simulink library "body_chassis_vert"  (R2018b)
settings: Solver=ode45  StartTime=0.0  StopTime=10.0  RelTol=1e-3  EnableMultiTasking=on
undefined symbols (not defined in the file): DiscIntNeverNeededParam, par_VEH, phi0, psip0, stepsize, v0
libraries: $bdroot x4
(part 1 of 2)
settings Model: Creator=CA-Win7Pro2  LastModifiedBy=ga35gug
settings DataIOCC: LimitDataPoints=on  SaveFormat=Array  SignalLoggingSaveFormat=ModelDataLogs
settings OptimizationCC: LifeSpan=inf
settings DebuggingCC: UnderspecifiedInitializationDetection=Classic  MergeDetectMultiDrivingBlocksExec=none  SolverPrmCheckMsg=warning  MultiTaskDSMMsg=warning  MultiTaskCondExecSysMsg=none  AllowSymbolicDim=off  SFUnexpectedBacktrackingDiag=warning  SFNoUnconditionalDefaultTransitionDiag=warning  SFExecutionAtInitializationDiag=none
settings HardwareCC: ProdBitPerPointer=32  ProdBitPerSizeT=32  ProdBitPerPtrDiffT=32  ProdLargestAtomicFloat=None  ProdIntDivRoundTo=Undefined  ProdEndianess=Unspecified  ProdWordSize=32  ProdHWDeviceType=32-bit Generic
settings ModelReferenceCC: PropagateSignalLabelsOutOfModel=off
settings SFSimCC: SimUseLocalCustomCode=off
settings RTWCC: RTWUseLocalCustomCode=off
settings CodeAppCC: StateflowObjectComments=on
settings GRTTargetCC: TargetLangStandard=C89/C90 (ANSI)  GeneratePreprocessorConditionals=Disable all
settings ConfigComp: CovMetricSettings=dw  CovHtmlReporting=on  CovSaveCumulativeToWorkspaceVar=on  CovSaveSingleToWorkspaceVar=on  CovExternalEMLEnable=off

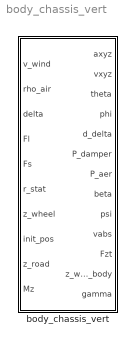
== system body_chassis_vert ==
  body_chassis_vert : Subsystem

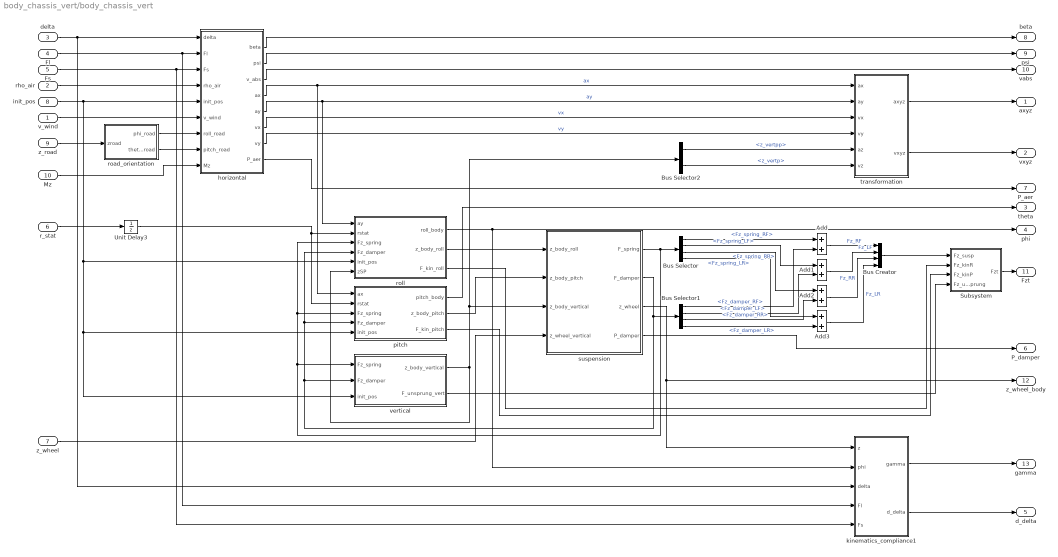
== system body_chassis_vert/body_chassis_vert ==
  v_wind : Inport
  rho_air : Inport  Port=2
  delta : Inport  Port=3
  Fl : Inport  Port=4
  Fs : Inport  Port=5
  r_stat : Inport  Port=6
  z_wheel : Inport  Port=7
  init_pos : Inport  Port=8
  z_road : Inport  Port=9
  Mz : Inport  Port=10
  Add{,1..3} (4 alike) : Sum
  Bus Creator : BusCreator  Inputs=4
  Bus Selector : BusSelector  OutputSignals=Fz_spring_RF,Fz_spring_LF,Fz_spring_RR,Fz_spring_LR
  Bus Selector1 : BusSelector  OutputSignals=Fz_damper_RF,Fz_damper_LF,Fz_damper_RR,Fz_damper_LR
  Bus Selector2 : BusSelector  OutputSignals=z_vertpp,z_vertp
  Subsystem : Subsystem
  Unit Delay3 : UnitDelay  SampleTime=-1
  horizontal : Subsystem
  kinematics_compliance1 : Subsystem
  pitch : Subsystem
  road_orientation : Subsystem
  roll : Subsystem
  suspension : Subsystem
  transformation : Subsystem
  vertical : Subsystem
  axyz : Outport
  vxyz : Outport  Port=2
  theta : Outport  Port=3
  phi : Outport  Port=4
  d_delta : Outport  Port=5
  P_damper : Outport  Port=6
  P_aer : Outport  Port=7
  beta : Outport  Port=8
  psi : Outport  Port=9
  vabs : Outport  Port=10
  Fzt : Outport  Port=11
  z_wheel_body : Outport  Port=12
  gamma : Outport  Port=13
  wires:
  Mz/1 -> horizontal/9(Mz)
  kinematics_compliance1/2(d_delta) -> d_delta/1
  kinematics_compliance1/1(gamma) -> gamma/1
  road_orientation/2(theta_road) -> horizontal/8(pitch_road)
  road_orientation/1(phi_road) -> horizontal/7(roll_road)
  z_road/1 -> road_orientation/1(zroad)
  suspension/3(z_wheel) -> z_wheel_body/1, kinematics_compliance1/1(z)
  roll/1(roll_body) -> phi/1, kinematics_compliance1/2(phi)
  suspension/1(F_spring) -> roll/3(Fz_spring), pitch/3(Fz_spring), vertical/1(Fz_spring), Bus Selector/1
  suspension/2(F_damper) -> roll/4(Fz_damper), pitch/4(Fz_damper), vertical/2(Fz_damper), Bus Selector1/1
  pitch/3(F_kin_pitch) -> Subsystem/3(Fz_kinP)
  roll/3(F_kin_roll) -> Subsystem/2(Fz_kinR)
  Subsystem/1(Fzt) -> Fzt/1
  Bus Creator/1 -> Subsystem/1(Fz_susp)
  pitch/1(pitch_body) -> theta/1
  horizontal/6(vx) -> transformation/3(vx)  "vx"
  horizontal/7(vy) -> transformation/4(vy)  "vy"
  horizontal/5(ay) -> transformation/2(ay), roll/1(ay)  "ay"
  horizontal/4(ax) -> transformation/1(ax), pitch/1(ax)  "ax"
  transformation/1(axyz) -> axyz/1
  transformation/2(vxyz) -> vxyz/1
  Bus Selector2/2 -> transformation/6(vz)  "<z_vertp>"
  Bus Selector2/1 -> transformation/5(az)  "<z_vertpp>"
  Add3/1 -> Bus Creator/4  "Fz_LR"
  Add2/1 -> Bus Creator/3  "Fz_RR"
  Add1/1 -> Bus Creator/2  "Fz_LF"
  Add/1 -> Bus Creator/1  "Fz_RF"
  Bus Selector1/4 -> Add3/2  "<Fz_damper_LR>"
  Bus Selector/4 -> Add3/1  "<Fz_spring_LR>"
  Bus Selector1/3 -> Add2/2  "<Fz_damper_RR>"
  Bus Selector/3 -> Add2/1  "<Fz_spring_RR>"
  Bus Selector1/2 -> Add1/2  "<Fz_damper_LF>"
  Bus Selector/2 -> Add1/1  "<Fz_spring_LF>"
  Bus Selector1/1 -> Add/2  "<Fz_damper_RF>"
  Bus Selector/1 -> Add/1  "<Fz_spring_RF>"
  roll/2(z_body_roll) -> suspension/1(z_body_roll)
  pitch/2(z_body_pitch) -> suspension/2(z_body_pitch)
  z_wheel/1 -> suspension/4(z_wheel_vertical)
  vertical/1(z_body_vertical) -> Bus Selector2/1, suspension/3(z_body_vertical), roll/6(zSP)
  v_wind/1 -> horizontal/6(v_wind)
  init_pos/1 -> horizontal/5(init_pos), pitch/5(init_pos), vertical/3(init_pos), roll/5(init_pos)
  rho_air/1 -> horizontal/4(rho_air)
  Unit Delay3/1 -> pitch/2(rstat), roll/2(rstat)
  delta/1 -> horizontal/1(delta), kinematics_compliance1/3(delta)
  horizontal/1(beta) -> beta/1
  horizontal/2(psi) -> psi/1
  Fl/1 -> horizontal/2(Fl), kinematics_compliance1/4(Fl)
  horizontal/3(v_abs) -> vabs/1
  Fs/1 -> horizontal/3(Fs), kinematics_compliance1/5(Fs)
  r_stat/1 -> Unit Delay3/1
  suspension/4(P_damper) -> P_damper/1
  horizontal/8(P_aer) -> P_aer/1
  vertical/2(F_unsprung_vert) -> Subsystem/4(Fz_unsprung)

== system body_chassis_vert/body_chassis_vert/Subsystem ==
  Fz_susp : Inport
  Fz_kinR : Inport  Port=2
  Fz_kinP : Inport  Port=3
  Fz_unsprung : Inport  Port=4
  Bus Creator : BusCreator  Inputs=4
  Bus Selector : BusSelector  OutputSignals=Fz_RF,Fz_LF,Fz_RR,Fz_LR
  Bus Selector1 : BusSelector  OutputSignals=F_kinR_RF,F_kinR_LF,F_kinR_RR,F_kinR_LR
  Bus Selector2 : BusSelector  OutputSignals=F_kinP_RF,F_kinP_LF,F_kinP_RR,F_kinP_LR
  Bus Selector3 : BusSelector  OutputSignals=F_us_RF,F_us_LF,F_us_RR,F_us_LR
  LF : Sum  Inputs=++++
  LR : Sum  Inputs=++++
  RF : Sum  Inputs=++++
  RR : Sum  Inputs=++++
  Fzt : Outport
  wires:
  Bus Selector2/4 -> LR/3  "<F_kinP_LR>"
  Bus Selector2/3 -> RR/3  "<F_kinP_RR>"
  Bus Creator/1 -> Fzt/1
  LR/1 -> Bus Creator/4  "Fz_LR"
  RR/1 -> Bus Creator/3  "Fz_RR"
  LF/1 -> Bus Creator/2  "Fz_LF"
  RF/1 -> Bus Creator/1  "Fz_RF"
  Bus Selector2/2 -> LF/3  "<F_kinP_LF>"
  Bus Selector2/1 -> RF/3  "<F_kinP_RF>"
  Bus Selector1/4 -> LR/2  "<F_kinR_LR>"
  Bus Selector1/3 -> RR/2  "<F_kinR_RR>"
  Bus Selector1/2 -> LF/2  "<F_kinR_LF>"
  Bus Selector1/1 -> RF/2  "<F_kinR_RF>"
  Bus Selector/4 -> LR/1  "<Fz_LR>"
  Bus Selector/3 -> RR/1  "<Fz_RR>"
  Bus Selector/2 -> LF/1  "<Fz_LF>"
  Bus Selector/1 -> RF/1  "<Fz_RF>"
  Fz_kinP/1 -> Bus Selector2/1
  Fz_kinR/1 -> Bus Selector1/1
  Fz_susp/1 -> Bus Selector/1
  Fz_unsprung/1 -> Bus Selector3/1
  Bus Selector3/1 -> RF/4  "<F_us_RF>"
  Bus Selector3/2 -> LF/4  "<F_us_LF>"
  Bus Selector3/3 -> RR/4  "<F_us_RR>"
  Bus Selector3/4 -> LR/4  "<F_us_LR>"

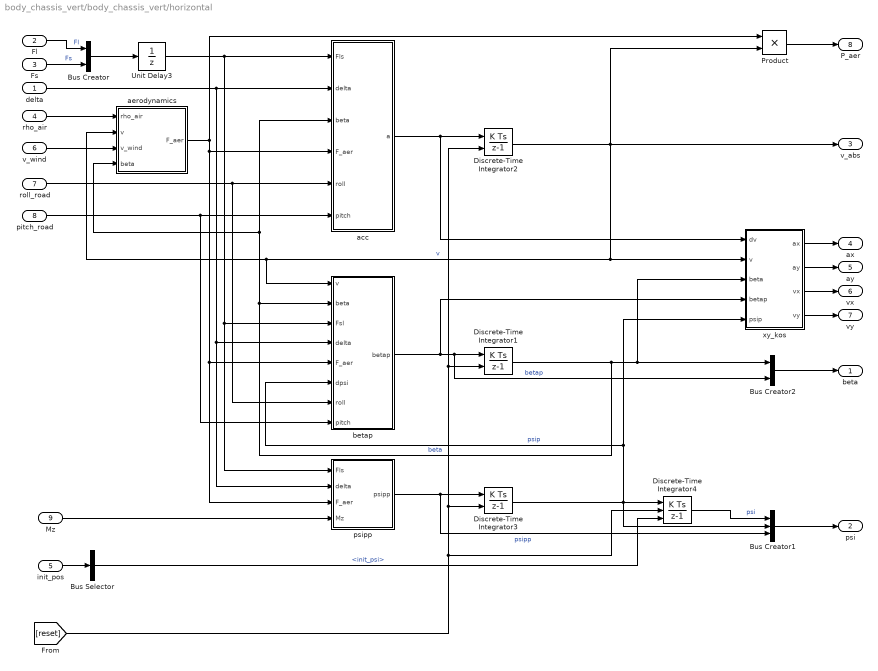
== system body_chassis_vert/body_chassis_vert/horizontal ==
  delta : Inport
  Fl : Inport  Port=2
  Fs : Inport  Port=3
  rho_air : Inport  Port=4
  init_pos : Inport  Port=5
  v_wind : Inport  Port=6
  roll_road : Inport  Port=7
  pitch_road : Inport  Port=8
  Mz : Inport  Port=9
  Bus Creator : BusCreator  Inputs=2
  Bus Creator1 : BusCreator  Inputs=3
  Bus Creator2 : BusCreator  Inputs=2
  Bus Selector : BusSelector  OutputSignals=init_psi
  Discrete-Time Integrator1 : DiscreteIntegrator  ExternalReset=sampled level  SampleTime=-1  ICPrevOutput=DiscIntNeverNeededParam  ICPrevScaledInput=DiscIntNeverNeededParam
  Discrete-Time Integrator2 : DiscreteIntegrator  ExternalReset=sampled level  InitialCondition=v0  SampleTime=-1  ICPrevOutput=DiscIntNeverNeededParam  ICPrevScaledInput=DiscIntNeverNeededParam
  Discrete-Time Integrator3 : DiscreteIntegrator  ExternalReset=sampled level  InitialCondition=psip0  SampleTime=-1  ICPrevOutput=DiscIntNeverNeededParam  ICPrevScaledInput=DiscIntNeverNeededParam
  Discrete-Time Integrator4 : DiscreteIntegrator  ExternalReset=sampled level  InitialConditionSource=external  SampleTime=-1  ICPrevOutput=DiscIntNeverNeededParam  ICPrevScaledInput=DiscIntNeverNeededParam
  Product : Product
  Unit Delay3 : UnitDelay  SampleTime=-1
  acc : Subsystem
  aerodynamics : Subsystem
  betap : Subsystem
  psipp : Subsystem
  xy_kos : Subsystem
  beta : Outport
  psi : Outport  Port=2
  v_abs : Outport  Port=3
  ax : Outport  Port=4
  ay : Outport  Port=5
  vx : Outport  Port=6
  vy : Outport  Port=7
  P_aer : Outport  Port=8
  wires:
  Mz/1 -> psipp/4(Mz)
  Bus Creator2/1 -> beta/1
  pitch_road/1 -> betap/8(pitch), acc/6(pitch)
  roll_road/1 -> acc/5(roll), betap/7(roll)
  xy_kos/4(vy) -> vy/1
  xy_kos/2(ay) -> ay/1
  v_wind/1 -> aerodynamics/3(v_wind)
  Bus Selector/1 -> Discrete-Time Integrator4/3  "<init_psi>"
  init_pos/1 -> Bus Selector/1
  [reset] -> Discrete-Time Integrator4/2, Discrete-Time Integrator3/2, Discrete-Time Integrator1/2, Discrete-Time Integrator2/2
  rho_air/1 -> aerodynamics/1(rho_air)
  xy_kos/1(ax) -> ax/1
  Bus Creator/1 -> Unit Delay3/1
  Fl/1 -> Bus Creator/1  "Fl"
  Fs/1 -> Bus Creator/2  "Fs"
  Discrete-Time Integrator3/1 -> xy_kos/5(psip), betap/6(dpsi), Discrete-Time Integrator4/1, Bus Creator1/2  "psip"
  psipp/1(psipp) -> Discrete-Time Integrator3/1, Bus Creator1/3  "psipp"
  Discrete-Time Integrator1/1 -> xy_kos/3(beta), Bus Creator2/1, aerodynamics/4(beta), acc/3(beta), betap/2(beta)  "beta"
  betap/1(betap) -> xy_kos/4(betap), Discrete-Time Integrator1/1, Bus Creator2/2  "betap"
  delta/1 -> acc/2(delta), psipp/2(delta), betap/4(delta)
  aerodynamics/1(F_aer) -> psipp/3(F_aer), betap/5(F_aer), acc/4(F_aer), Product/1
  Discrete-Time Integrator2/1 -> v_abs/1, Product/2, aerodynamics/2(v), betap/1(v), xy_kos/2(v)  "v"
  acc/1(a) -> xy_kos/1(dv), Discrete-Time Integrator2/1
  Discrete-Time Integrator4/1 -> Bus Creator1/1  "psi"
  Bus Creator1/1 -> psi/1
  xy_kos/3(vx) -> vx/1
  Unit Delay3/1 -> acc/1(Fls), psipp/1(Fls), betap/3(Fsl)
  Product/1 -> P_aer/1

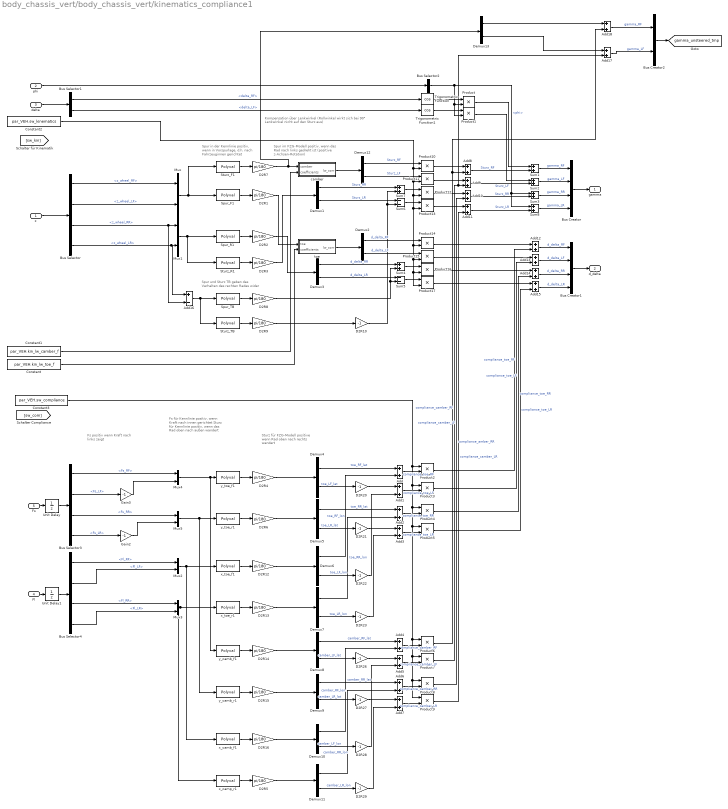
== system body_chassis_vert/body_chassis_vert/kinematics_compliance1 ==
  note: Spur und Sturz TB geben das
      | Verhalten des rechten Rades wider
  note: Spur in der Kennlinie positiv,
      | wenn in Vorspurlage, d.h. nach
      | Fahrzeuginnen gerichtet
  note: Fs für Kennlinie positiv,
      | wenn Kraft nach innen gerichtet
      |
      | Sturz für Kennlinie positiv,
      | wenn das Rad oben nach
      | außen wandert
  note: Fs positiv wenn
      | Kraft nach links zeigt
  note: Kompensation über Lenkwinkel
      | (Rollwinkel wirkt sich bei 90° Lenkwinkel nicht auf den Sturz aus)
  note: Sturz für FZG-Modell
      | positive wenn Rad oben
      | nach rechts wandert
  note: Spur im FZG-Modell positiv,
      | wenn das Rad nach links gedreht ist
      | (positive z-Achsen-Rotation)
  z : Inport
  phi : Inport  Port=2
  delta : Inport  Port=3
  Fl : Inport  Port=4
  Fs : Inport  Port=5
  Add{,1..15,17..18} (18 alike) : Sum
  Add16 : Sum  Inputs=+-
  Bus Creator : BusCreator  Inputs=4
  Bus Creator1 : BusCreator  Inputs=4
  Bus Creator2 : BusCreator  Inputs=2
  Bus Selector : BusSelector  OutputSignals=z_wheel_RF,z_wheel_LF,z_wheel_RR,z_wheel_LR
  Bus Selector1 : BusSelector  OutputSignals=delta_RF,delta_LF
  Bus Selector2 : BusSelector  OutputSignals=phi
  Bus Selector3 : BusSelector  OutputSignals=Fs_RF,Fs_LF,Fs_RR,Fs_LR
  Bus Selector4 : BusSelector  OutputSignals=Fl_RF,Fl_LF,Fl_RR,Fl_LR
  Constant : Constant  Value=par_VEH.kin_lw_toe_f
  Constant1 : Constant  Value=par_VEH.kin_lw_camber_f
  Constant2 : Constant  Value=par_VEH.sw_kinematics
  Constant3 : Constant  Value=par_VEH.sw_compliance
  D2R{1..9,12..16} (14 alike) : Gain  Gain=pi/180
  D2R{10,20..23,26..29} (9 alike) : Gain  Gain=-1
  Demux{1..13} (13 alike) : Demux  Outputs=2
  Gain2 : Gain  Gain=-1
  Gain3 : Gain  Gain=-1
  Mux{,1..5} (6 alike) : Mux  Inputs=2
  Product{,1..17} (18 alike) : Product  RndMeth=Zero
  Spur_F1 : Polyval  Coefs=par_VEH.kin_toe_f
  Spur_R1 : Polyval  Coefs=par_VEH.kin_toe_r
  Spur_TB : Polyval  Coefs=par_VEH.elkin_toe_twistbeam
  Sturz_F1 : Polyval  Coefs=par_VEH.kin_camb_f
  Sturz_R1 : Polyval  Coefs=par_VEH.kin_camb_r
  Sturz_TB : Polyval  Coefs=par_VEH.elkin_camb_twistbeam
  Sum{1..4,7..8} (6 alike) : Sum
  Sum5 : Sum  Inputs=--
  Sum6 : Sum  Inputs=--
  Trigonometric Function : Trigonometry  Operator=cos
  Trigonometric Function1 : Trigonometry  Operator=cos
  Unit Delay : UnitDelay  SampleTime=-1
  Unit Delay1 : UnitDelay  SampleTime=-1
  camber : Subsystem
  toe : Subsystem
  x_camb_f1 : Polyval  Coefs=par_VEH.elkin_x_camb_f
  x_camp_r1 : Polyval  Coefs=par_VEH.elkin_x_camb_r
  x_toe_f1 : Polyval  Coefs=par_VEH.elkin_x_toe_f
  x_toe_r1 : Polyval  Coefs=par_VEH.elkin_x_toe_r
  y_camb_f1 : Polyval  Coefs=par_VEH.elkin_y_camb_f
  y_camb_r1 : Polyval  Coefs=par_VEH.elkin_y_camb_r
  y_toe_f1 : Polyval  Coefs=par_VEH.elkin_y_toe_f
  y_toe_r1 : Polyval  Coefs=par_VEH.elkin_y_toe_r
  gamma : Outport
  d_delta : Outport  Port=2
  tag scope: gamma_unsteered_tmp=global
  wires:
  Bus Creator2/1 -> [gamma_unsteered_tmp]
  Add17/1 -> Bus Creator2/2  "gamma_LF"
  Add18/1 -> Bus Creator2/1  "gamma_RF"
  Demux13/1 -> Add18/1
  Demux13/2 -> Add17/1
  Constant1/1 -> camber/2(coefficients)
  Constant/1 -> toe/2(coefficients)
  D2R1/1 -> toe/1("toe ")
  toe/1(lw_corr) -> Demux2/1
  camber/1(lw_corr) -> Demux12/1
  Mux1/1 -> Sturz_R1/1, Spur_R1/1
  Spur_R1/1 -> D2R2/1
  Spur_F1/1 -> D2R1/1
  Sturz_F1/1 -> D2R7/1
  D2R7/1 -> camber/1("camber "), Demux13/1
  Mux/1 -> Sturz_F1/1, Spur_F1/1
  y_toe_f1/1 -> D2R4/1
  y_toe_r1/1 -> D2R6/1
  x_toe_f1/1 -> D2R12/1
  x_toe_r1/1 -> D2R13/1
  y_camb_f1/1 -> D2R14/1
  y_camb_r1/1 -> D2R15/1
  x_camb_f1/1 -> D2R16/1
  x_camp_r1/1 -> D2R5/1
  D2R3/1 -> Demux1/1
  Demux2/1 -> Product14/1  "d_delta_RF"
  Demux3/1 -> Sum4/1  "d_delta_RR"
  Add7/1 -> Product9/2  "compliance_camber_LR"
  Add6/1 -> Product8/2  "compliance_camber_RR"
  Add5/1 -> Product7/2  "compliance_camber_LF"
  Add4/1 -> Product6/2  "compliance_camber_RF"
  Add3/1 -> Product5/2  "compliance_toe_LR"
  Add2/1 -> Product4/2  "compliance_toe_RR"
  Add1/1 -> Product3/2  "compliance_toe_LF"
  Add/1 -> Product2/2  "compliance_toe_RF"
  Add13/1 -> Bus Creator1/2  "d_delta_LF"
  Unit Delay1/1 -> Bus Selector4/1
  Unit Delay/1 -> Bus Selector3/1
  Fs/1 -> Unit Delay/1
  Fl/1 -> Unit Delay1/1
  Bus Selector3/1 -> Mux4/1  "<Fs_RF>"
  Bus Selector3/2 -> Gain3/1  "<Fs_LF>"
  Bus Selector3/3 -> Mux5/1  "<Fs_RR>"
  Bus Selector3/4 -> Gain2/1  "<Fs_LR>"
  Bus Selector4/1 -> Mux2/1  "<Fl_RF>"
  Bus Selector4/2 -> Mux2/2  "<Fl_LF>"
  Bus Selector4/3 -> Mux3/1  "<Fl_RR>"
  Bus Selector4/4 -> Mux3/2  "<Fl_LR>"
  Mux2/1 -> x_toe_f1/1, x_camb_f1/1
  Mux3/1 -> x_camp_r1/1, x_toe_r1/1
  Mux4/1 -> y_toe_f1/1, y_camb_f1/1
  Mux5/1 -> y_toe_r1/1, y_camb_r1/1
  D2R4/1 -> Demux4/1
  D2R6/1 -> Demux5/1
  D2R12/1 -> Demux6/1
  D2R13/1 -> Demux7/1
  D2R14/1 -> Demux8/1
  D2R15/1 -> Demux9/1
  D2R16/1 -> Demux10/1
  D2R5/1 -> Demux11/1
  Demux4/1 -> Add/1  "toe_RF_lat"
  Demux4/2 -> D2R20/1  "toe_LF_lat"
  Demux5/1 -> Add2/1  "toe_RR_lat"
  Demux5/2 -> D2R21/1  "toe_LR_lat"
  Demux6/1 -> Add/2  "toe_RF_lon"
  Demux6/2 -> D2R22/1  "toe_LF_lon"
  Demux7/1 -> Add2/2  "toe_RR_lon"
  Demux7/2 -> D2R23/1  "toe_LR_lon"
  Demux8/1 -> Add4/1  "camber_RF_lat"
  Demux8/2 -> D2R26/1  "camber_LF_lat"
  Demux9/1 -> Add6/1  "camber_RR_lat"
  Demux9/2 -> D2R27/1  "camber_LR_lat"
  Demux10/1 -> Add4/2  "camber_RF_lon"
  Demux10/2 -> D2R28/1  "camber_LF_lon"
  Demux11/1 -> Add6/2  "camber_RR_lon"
  Demux11/2 -> D2R29/1  "camber_LR_lon"
  delta/1 -> Bus Selector1/1
  Demux1/2 -> Sum6/1  "Sturz_LR"
  D2R2/1 -> Demux3/1
  Bus Creator1/1 -> d_delta/1
  Bus Creator/1 -> gamma/1
  Demux12/2 -> Product11/1  "Sturz_LF"
  Sturz_R1/1 -> D2R3/1
  z/1 -> Bus Selector/1
  phi/1 -> Bus Selector2/1
  Bus Selector2/1 -> Product1/2, Product/2, Sum3/1, Sum8/1  "<phi>"
  Gain2/1 -> Mux5/2
  D2R20/1 -> Add1/1
  D2R21/1 -> Add3/1
  D2R23/1 -> Add3/2
  Spur_TB/1 -> D2R8/1
  Demux3/2 -> Sum5/1  "d_delta_LR"
  Add16/1 -> Spur_TB/1, Sturz_TB/1
  Sturz_TB/1 -> D2R9/1
  Demux1/1 -> Sum7/1  "Sturz_RR"
  D2R9/1 -> D2R10/1
  D2R10/1 -> Sum6/2, Sum7/2
  D2R8/1 -> Sum5/2, Sum4/2
  Constant3/1 -> Product9/1, Product8/1, Product7/1, Product6/1, Product5/1, Product4/1, Product3/1, Product2/1
  Bus Selector/1 -> Mux/1  "<z_wheel_RF>"
  Bus Selector/2 -> Mux/2  "<z_wheel_LF>"
  Bus Selector/3 -> Add16/2, Mux1/1  "<z_wheel_RR>"
  Bus Selector/4 -> Mux1/2, Add16/1  "<z_wheel_LR>"
  Add9/1 -> Sum2/2  "Sturz_LF"
  Trigonometric Function1/1 -> Product1/1
  Trigonometric Function/1 -> Product/1
  Product/1 -> Sum1/1
  Product1/1 -> Sum2/1
  Add10/1 -> Sum3/2  "Sturz_RR"
  Add11/1 -> Sum8/2  "Sturz_LR"
  Sum8/1 -> Bus Creator/4  "gamma_LR"
  Sum3/1 -> Bus Creator/3  "gamma_RR"
  Sum2/1 -> Bus Creator/2  "gamma_LF"
  Sum1/1 -> Bus Creator/1  "gamma_RF"
  Demux12/1 -> Product10/1  "Sturz_RF"
  Sum6/1 -> Product13/1
  Demux2/2 -> Product15/1  "d_delta_LF"
  Sum4/1 -> Product16/1
  Sum5/1 -> Product17/1
  Constant2/1 -> Product14/2, Product15/2, Product17/2, Product16/2, Product13/2, Product12/2, Product11/2, Product10/2
  Product10/1 -> Add8/1
  Product11/1 -> Add9/1
  Product12/1 -> Add10/1
  Product13/1 -> Add11/1
  Product14/1 -> Add12/1
  Product15/1 -> Add13/1
  Product16/1 -> Add14/1
  Product17/1 -> Add15/1
  Add15/1 -> Bus Creator1/4  "d_delta_LR"
  Add12/1 -> Bus Creator1/1  "d_delta_RF"
  Add14/1 -> Bus Creator1/3  "d_delta_RR"
  Gain3/1 -> Mux4/2
  Add8/1 -> Sum1/2  "Sturz_RF"
  Product2/1 -> Add12/2  "compliance_toe_RF"
  Product3/1 -> Add13/2  "compliance_toe_LF"
  Product4/1 -> Add14/2  "compliance_toe_RR"
  Product5/1 -> Add15/2  "compliance_toe_LR"
  Product6/1 -> Add8/2, Add18/2  "compliance_camber_RF"
  Product7/1 -> Add9/2, Add17/2  "compliance_camber_LF"
  Product8/1 -> Add10/2  "compliance_amber_RR"
  Product9/1 -> Add11/2  "compliance_camber_LR"
  D2R22/1 -> Add1/2
  Bus Selector1/2 -> Trigonometric Function1/1  "<delta_LF>"
  Bus Selector1/1 -> Trigonometric Function/1  "<delta_RF>"
  Sum7/1 -> Product12/1
  D2R26/1 -> Add5/1
  D2R27/1 -> Add7/1
  D2R28/1 -> Add5/2
  D2R29/1 -> Add7/2

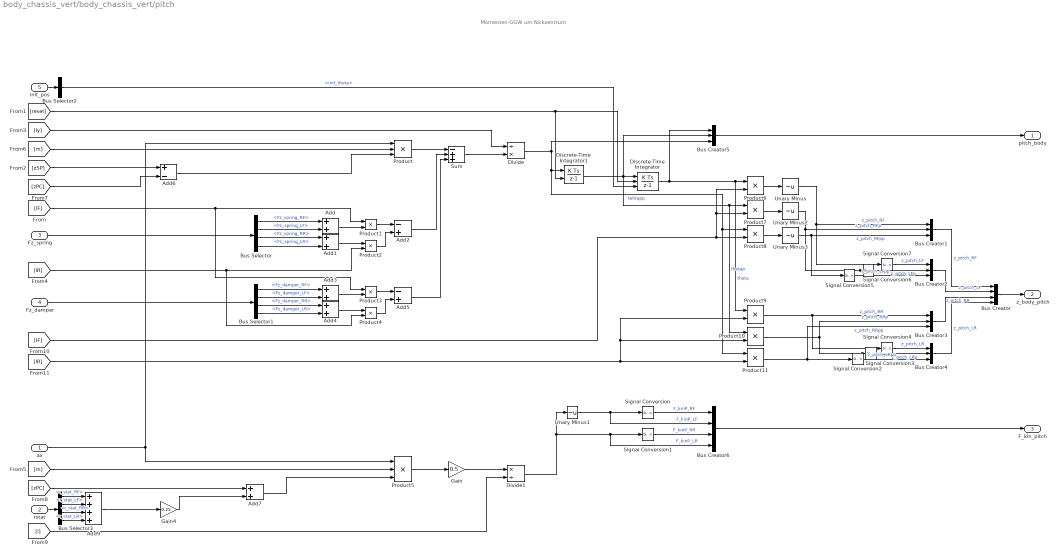
== system body_chassis_vert/body_chassis_vert/pitch ==
  note: Momenten-GGW um Nickzentrum
  ax : Inport
  rstat : Inport  Port=2
  Fz_spring : Inport  Port=3
  Fz_damper : Inport  Port=4
  init_pos : Inport  Port=5
  Add{,1,3..4,7} (5 alike) : Sum
  Add2 : Sum  Inputs=-+
  Add5 : Sum  Inputs=-+
  Add6 : Sum  Inputs=+-
  Add9 : Sum  Inputs=++++
  Bus Creator : BusCreator  Inputs=4
  Bus Creator{1..5} (5 alike) : BusCreator  Inputs=3
  Bus Creator6 : BusCreator  Inputs=4
  Bus Selector : BusSelector  OutputSignals=Fz_spring_RF,Fz_spring_LF,Fz_spring_RR,Fz_spring_LR
  Bus Selector1 : BusSelector  OutputSignals=Fz_damper_RF,Fz_damper_LF,Fz_damper_RR,Fz_damper_LR
  Bus Selector2 : BusSelector  OutputSignals=init_theta
  Bus Selector3 : BusSelector  OutputSignals=r_stat_RF,r_stat_LF,r_stat_RR,r_stat_LR
  Discrete-Time Integrator : DiscreteIntegrator  ExternalReset=sampled level  InitialConditionSource=external  SampleTime=stepsize  ICPrevOutput=DiscIntNeverNeededParam  ICPrevScaledInput=DiscIntNeverNeededParam
  Discrete-Time Integrator1 : DiscreteIntegrator  ExternalReset=sampled level  SampleTime=stepsize  ICPrevOutput=DiscIntNeverNeededParam  ICPrevScaledInput=DiscIntNeverNeededParam
  Divide : Product  Inputs=/*
  Divide1 : Product  Inputs=*/
  Gain : Gain  Gain=0.5
  Gain4 : Gain  Gain=0.25
  Product : Product  Inputs=3  RndMeth=Zero
  Product{1..4,6..11} (10 alike) : Product  RndMeth=Zero
  Product5 : Product  Inputs=3  RndMeth=Zero
  Signal Conversion{,1..7} (8 alike) : SignalConversion  OverrideOpt=off
  Sum : Sum  Inputs=-++
  Unary Minus{,1..3} (4 alike) : UnaryMinus
  pitch_body : Outport
  z_body_pitch : Outport  Port=2
  F_kin_pitch : Outport  Port=3
  wires:
  Unary Minus1/1 -> Signal Conversion/1, Bus Creator6/2  "F_kinP_LF"
  ax/1 -> Product/1, Product5/1
  Divide1/1 -> Unary Minus1/1, Bus Creator6/4, Signal Conversion1/1  "F_kinP_LR"
  Signal Conversion7/1 -> Bus Creator2/1  "z_pitch_LF"
  Signal Conversion6/1 -> Bus Creator2/2  "z_pitch_LFp"
  Signal Conversion5/1 -> Bus Creator2/3  "z_pitch_LFpp"
  Signal Conversion4/1 -> Bus Creator4/1  "z_pitch_LR"
  Signal Conversion3/1 -> Bus Creator4/2  "z_pitch_LRp"
  Signal Conversion2/1 -> Bus Creator4/3  "z_pitch_LRpp"
  Gain4/1 -> Add7/2
  rstat/1 -> Bus Selector3/1
  Bus Selector3/4 -> Add9/4  "<r_stat_LR>"
  Bus Selector3/3 -> Add9/3  "<r_stat_RR>"
  Bus Selector3/2 -> Add9/2  "<r_stat_LF>"
  Bus Selector3/1 -> Add9/1  "<r_stat_RF>"
  Add9/1 -> Gain4/1
  [zPC] -> Add7/1
  [zPC] -> Add6/2
  [zSP] -> Add6/1
  [reset] -> Discrete-Time Integrator/2, Discrete-Time Integrator1/2
  Bus Selector2/1 -> Discrete-Time Integrator/3  "<init_theta>"
  init_pos/1 -> Bus Selector2/1
  Bus Creator/1 -> z_body_pitch/1
  Bus Creator1/1 -> Bus Creator/1  "z_pitch_RF"
  Bus Creator2/1 -> Bus Creator/2  "z_pitch_LF"
  Bus Creator3/1 -> Bus Creator/3  "z_pitch_RR"
  Bus Creator4/1 -> Bus Creator/4  "z_pitch_LR"
  Unary Minus2/1 -> Bus Creator1/2, Signal Conversion6/1  "z_pitch_RFp"
  Discrete-Time Integrator/1 -> Bus Creator5/1, Product9/1, Product6/1  "theta"
  Bus Creator5/1 -> pitch_body/1
  [m] -> Product/2
  Sum/1 -> Divide/2
  [Iy] -> Divide/1
  Divide/1 -> Product8/1, Product11/1, Discrete-Time Integrator1/1, Bus Creator5/3  "tehtapp"
  Discrete-Time Integrator1/1 -> Discrete-Time Integrator/1, Product10/1, Product7/1, Bus Creator5/2  "thetap"
  Fz_spring/1 -> Bus Selector/1
  Bus Selector/1 -> Add/1  "<Fz_spring_RF>"
  Bus Selector/2 -> Add/2  "<Fz_spring_LF>"
  Bus Selector/3 -> Add1/1  "<Fz_spring_RR>"
  Bus Selector/4 -> Add1/2  "<Fz_spring_LR>"
  Fz_damper/1 -> Bus Selector1/1
  Add/1 -> Product1/2
  Add1/1 -> Product2/1
  Product1/1 -> Add2/1
  Product2/1 -> Add2/2
  Bus Selector1/1 -> Add3/1  "<Fz_damper_RF>"
  Bus Selector1/2 -> Add3/2  "<Fz_damper_LF>"
  Bus Selector1/3 -> Add4/1  "<Fz_damper_RR>"
  Bus Selector1/4 -> Add4/2  "<Fz_damper_LR>"
  Add3/1 -> Product3/2
  Add4/1 -> Product4/1
  Product3/1 -> Add5/1
  Product4/1 -> Add5/2
  Unary Minus/1 -> Bus Creator1/1, Signal Conversion7/1  "z_pitch_RF"
  Unary Minus3/1 -> Signal Conversion5/1, Bus Creator1/3  "z_pitch_RFpp"
  Add6/1 -> Product/3
  Product/1 -> Sum/1
  Add5/1 -> Sum/3
  Add2/1 -> Sum/2
  Add7/1 -> Product5/3
  Product5/1 -> Gain/1
  [l] -> Divide1/2
  Gain/1 -> Divide1/1
  Signal Conversion1/1 -> Bus Creator6/3  "F_kinP_RR"
  Bus Creator6/1 -> F_kin_pitch/1
  [m] -> Product5/2
  Signal Conversion/1 -> Bus Creator6/1  "F_kinP_RF"
  [lR] -> Product2/2, Product4/2
  [lF] -> Product1/1, Product3/1
  [lF] -> Product8/2, Product7/2, Product6/2
  [lR] -> Product9/2, Product10/2, Product11/2
  Product9/1 -> Signal Conversion4/1, Bus Creator3/1  "z_pitch_RR"
  Product10/1 -> Signal Conversion3/1, Bus Creator3/2  "z_pitch_RRp"
  Product11/1 -> Signal Conversion2/1, Bus Creator3/3  "z_pitch_RRpp"
  Product8/1 -> Unary Minus3/1
  Product6/1 -> Unary Minus/1
  Product7/1 -> Unary Minus2/1

== system body_chassis_vert/body_chassis_vert/road_orientation ==
  zroad : Inport
  Bus Selector1 : BusSelector  OutputSignals=zroad_RF,zroad_LF,zroad_RR,zroad_LR
  Divide7 : Product  Inputs=*/
  Divide8 : Product  Inputs=*/
  Gain{,1..4} (5 alike) : Gain  Gain=0.5
  Subtract{14..15,17..19} (5 alike) : Sum
  Subtract16 : Sum  Inputs=-+
  Subtract20 : Sum  Inputs=+-
  Trigonometric Function : Trigonometry  Operator=asin
  Trigonometric Function1 : Trigonometry  Operator=asin
  phi_road : Outport
  theta_road : Outport  Port=2
  wires:
  Divide8/1 -> Trigonometric Function/1
  [l] -> Divide8/2
  Subtract20/1 -> Divide8/1
  Gain4/1 -> Subtract20/2
  Gain3/1 -> Subtract20/1
  Subtract19/1 -> Gain4/1
  Subtract18/1 -> Gain3/1
  Bus Selector1/1 -> Subtract14/1, Subtract18/1  "<zroad_RF>"
  Trigonometric Function/1 -> theta_road/1
  Divide7/1 -> Trigonometric Function1/1
  Subtract17/1 -> Gain2/1
  Gain2/1 -> Divide7/2
  Subtract16/1 -> Divide7/1
  Gain1/1 -> Subtract16/2
  Gain/1 -> Subtract16/1
  Bus Selector1/4 -> Subtract15/2, Subtract19/2  "<zroad_LR>"
  Bus Selector1/2 -> Subtract15/1, Subtract18/2  "<zroad_LF>"
  Subtract15/1 -> Gain1/1
  Bus Selector1/3 -> Subtract14/2, Subtract19/1  "<zroad_RR>"
  [sR] -> Subtract17/1
  Subtract14/1 -> Gain/1
  Trigonometric Function1/1 -> phi_road/1
  [sF] -> Subtract17/2
  zroad/1 -> Bus Selector1/1

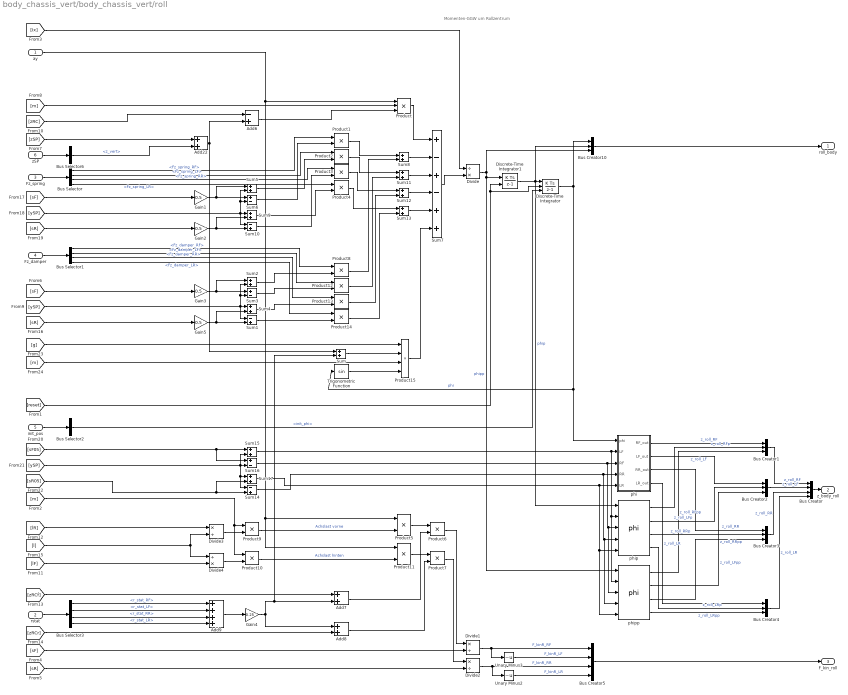
== system body_chassis_vert/body_chassis_vert/roll ==
  note: Momenten-GGW um Rollzentrum
  ay : Inport
  rstat : Inport  Port=2
  Fz_spring : Inport  Port=3
  Fz_damper : Inport  Port=4
  init_pos : Inport  Port=5
  zSP : Inport  Port=6
  Add22 : Sum
  Add6 : Sum  Inputs=-+
  Add7 : Sum
  Add8 : Sum
  Add9 : Sum  Inputs=++++
  Bus Creator : BusCreator  Inputs=4
  Bus Creator{1..4,10} (5 alike) : BusCreator  Inputs=3
  Bus Creator5 : BusCreator  Inputs=4
  Bus Selector : BusSelector  OutputSignals=Fz_spring_RF,Fz_spring_LF,Fz_spring_RR,Fz_spring_LR
  Bus Selector1 : BusSelector  OutputSignals=Fz_damper_RF,Fz_damper_LF,Fz_damper_RR,Fz_damper_LR
  Bus Selector2 : BusSelector  OutputSignals=init_phi
  Bus Selector3 : BusSelector  OutputSignals=r_stat_RF,r_stat_LF,r_stat_RR,r_stat_LR
  Bus Selector6 : BusSelector  OutputSignals=z_vert
  Discrete-Time Integrator : DiscreteIntegrator  ExternalReset=sampled level  InitialConditionSource=external  InitialCondition=phi0  SampleTime=stepsize  ICPrevOutput=DiscIntNeverNeededParam  ICPrevScaledInput=DiscIntNeverNeededParam
  Discrete-Time Integrator1 : DiscreteIntegrator  ExternalReset=sampled level  SampleTime=stepsize  ICPrevOutput=DiscIntNeverNeededParam  ICPrevScaledInput=DiscIntNeverNeededParam
  Divide : Product  Inputs=/*
  Divide1 : Product  Inputs=*/
  Divide2 : Product  Inputs=*/
  Divide3 : Product  Inputs=*/
  Divide4 : Product  Inputs=/*
  Gain{1..3,5} (4 alike) : Gain  Gain=0.5
  Gain4 : Gain  Gain=0.25
  Product : Product  Inputs=3  RndMeth=Zero
  Product{1..14} (14 alike) : Product  RndMeth=Zero
  Product15 : Product  Inputs=4
  Sum{,2,4..5,8..9,11..13,15,17} (11 alike) : Sum
  Sum1 : Sum  Inputs=-+
  Sum10 : Sum  Inputs=-+
  Sum14 : Sum  Inputs=-+
  Sum16 : Sum  Inputs=+-
  Sum3 : Sum  Inputs=+-
  Sum6 : Sum  Inputs=+-
  Sum7 : Sum  Inputs=+-+-++
  Trigonometric Function : Trigonometry
  Unary Minus2 : UnaryMinus
  Unary Minus3 : UnaryMinus
  phi : Subsystem
  phip : $bdroot/body_chassis_vert/roll/phi  SystemSampleTime=-1
  phipp : $bdroot/body_chassis_vert/roll/phi  SystemSampleTime=-1
  roll_body : Outport
  z_body_roll : Outport  Port=2
  F_kin_roll : Outport  Port=3
  wires:
  Product15/1 -> Sum7/6
  [m] -> Product15/3
  Trigonometric Function/1 -> Product15/4
  Sum/1 -> Product15/2
  [g] -> Product15/1
  [m] -> Product/2
  Sum17/1 -> phi/5(LR), phipp/5, phip/5
  Sum14/1 -> phipp/4, phip/4, phi/4(RR)
  Sum16/1 -> phi/3(RF), phipp/3, phip/3
  Sum15/1 -> phi/2(LF), phipp/2, phip/2
  [sR05] -> Sum14/2, Sum17/2
  [sF05] -> Sum16/1, Sum15/1
  Product14/1 -> Sum13/2
  Product13/1 -> Sum12/2
  Product12/1 -> Sum11/2
  Product8/1 -> Sum8/2
  Product4/1 -> Sum13/1
  Product3/1 -> Sum12/1
  Product2/1 -> Sum11/1
  Sum1/1 -> Product14/2
  Sum4/1 -> Product13/2
  Sum3/1 -> Product12/2
  Sum2/1 -> Product8/2
  Gain5/1 -> Sum1/2, Sum4/2
  Gain3/1 -> Sum3/1, Sum2/1
  [sR] -> Gain5/1
  [sF] -> Gain3/1
  Unary Minus3/1 -> Bus Creator5/2  "F_kinR_LF"
  Unary Minus2/1 -> Bus Creator5/4  "F_kinR_LR"
  Sum13/1 -> Sum7/5
  Product/1 -> Sum7/1
  Sum12/1 -> Sum7/4
  Sum11/1 -> Sum7/3
  Sum9/1 -> Product4/2
  Sum10/1 -> Product3/2
  Sum5/1 -> Product2/2
  Sum6/1 -> Product1/2
  Gain2/1 -> Sum9/2, Sum10/2
  Gain1/1 -> Sum5/1, Sum6/1
  Fz_damper/1 -> Bus Selector1/1
  Fz_spring/1 -> Bus Selector/1
  [sR] -> Gain2/1
  [sF] -> Gain1/1
  Bus Selector1/4 -> Product14/1  "<Fz_damper_LR>"
  Bus Selector1/3 -> Product13/1  "<Fz_damper_RR>"
  Bus Selector1/2 -> Product12/1  "<Fz_damper_LF>"
  Bus Selector1/1 -> Product8/1  "<Fz_damper_RF>"
  Bus Selector/4 -> Product4/1  "<Fz_spring_LR>"
  Bus Selector/2 -> Product2/1  "<Fz_spring_LF>"
  Bus Selector/3 -> Product3/1  "<Fz_spring_RR>"
  Bus Selector/1 -> Product1/1  "<Fz_spring_RF>"
  Product7/1 -> Divide2/1
  Product6/1 -> Divide1/1
  Gain4/1 -> Add7/2, Sum/2, Add8/1
  Bus Selector3/4 -> Add9/4  "<r_stat_LR>"
  Bus Selector3/3 -> Add9/3  "<r_stat_RR>"
  Bus Selector3/2 -> Add9/2  "<r_stat_LF>"
  Bus Selector3/1 -> Add9/1  "<r_stat_RF>"
  rstat/1 -> Bus Selector3/1
  Bus Selector2/1 -> Discrete-Time Integrator/3  "<init_phi>"
  init_pos/1 -> Bus Selector2/1
  Bus Creator10/1 -> roll_body/1
  Add8/1 -> Product7/2
  Product11/1 -> Product7/1
  Product5/1 -> Product6/1
  Product10/1 -> Product11/2  "Achslast hinten"
  Product9/1 -> Product5/2  "Achslast vorne"
  Divide4/1 -> Product10/2
  Divide3/1 -> Product9/2
  [l] -> Divide4/1, Divide3/2
  [zRCr] -> Add8/2
  [reset] -> Discrete-Time Integrator/2, Discrete-Time Integrator1/2
  Add9/1 -> Gain4/1
  [zRCf] -> Add7/1
  Add22/1 -> Sum/1, Add6/2
  [zRC] -> Add6/1
  Bus Creator/1 -> z_body_roll/1
  Bus Creator1/1 -> Bus Creator/1  "z_roll_RF"
  Bus Creator2/1 -> Bus Creator/2  "z_roll_LF"
  Bus Creator3/1 -> Bus Creator/3  "z_roll_RR"
  Bus Creator4/1 -> Bus Creator/4  "z_roll_LR"
  phi/1(RF_out) -> Bus Creator1/1  "z_roll_RF"
  phip/1 -> Bus Creator1/2  "z_roll_RFp"
  phipp/1 -> Bus Creator1/3  "z_roll_RFpp"
  phi/2(LF_out) -> Bus Creator2/1  "z_roll_LF"
  phip/2 -> Bus Creator2/2  "z_roll_LFp"
  phipp/2 -> Bus Creator2/3  "z_roll_LFpp"
  phi/3(RR_out) -> Bus Creator3/1  "z_roll_RR"
  phip/3 -> Bus Creator3/2  "z_roll_RRp"
  phipp/3 -> Bus Creator3/3  "z_roll_RRpp"
  phi/4(LR_out) -> Bus Creator4/1  "z_roll_LR"
  phip/4 -> Bus Creator4/2  "z_roll_LRp"
  phipp/4 -> Bus Creator4/3  "z_roll_LRpp"
  [Ix] -> Divide/1
  Divide/1 -> Bus Creator10/3, phipp/1, Discrete-Time Integrator1/1  "phipp"
  Discrete-Time Integrator1/1 -> phip/1, Bus Creator10/2, Discrete-Time Integrator/1  "phip"
  [sF] -> Divide1/2
  [sR] -> Divide2/2
  Divide1/1 -> Unary Minus3/1, Bus Creator5/1  "F_kinR_RF"
  Divide2/1 -> Unary Minus2/1, Bus Creator5/3  "F_kinR_RR"
  Bus Creator5/1 -> F_kin_roll/1
  [m] -> Product9/1, Product10/1
  Sum7/1 -> Divide/2
  ay/1 -> Product/1, Product5/1, Product11/1
  Product1/1 -> Sum8/1
  Sum8/1 -> Sum7/2
  [ySP] -> Sum1/1, Sum4/1, Sum3/2, Sum2/2
  [ySP] -> Sum5/2, Sum6/2, Sum9/1, Sum10/1
  [ySP] -> Sum16/2, Sum15/2, Sum14/1, Sum17/1
  Add7/1 -> Product6/2
  zSP/1 -> Bus Selector6/1
  [zSP] -> Add22/1
  Bus Selector6/1 -> Add22/2  "<z_vert>"
  [lR] -> Divide3/1
  [lF] -> Divide4/2
  Discrete-Time Integrator/1 -> Bus Creator10/1, Trigonometric Function/1, phi/1(phi)  "phi"
  Add6/1 -> Product/3

== system body_chassis_vert/body_chassis_vert/suspension ==
  z_body_roll : Inport
  z_body_pitch : Inport  Port=2
  z_body_vertical : Inport  Port=3
  z_wheel_vertical : Inport  Port=4
  Add{,1..3} (4 alike) : Sum
  Bus Creator : BusCreator  Inputs=4
  Bus Selector : BusSelector  OutputSignals=Fz_spring_RF,Fz_spring_LF,Fz_spring_RR,Fz_spring_LR
  Bus Selector1 : BusSelector  OutputSignals=Fz_arb_RF,Fz_arb_LF,Fz_arb_RR,Fz_arb_LR
  arb : Subsystem
  damper : Subsystem
  spring : Subsystem
  F_spring : Outport
  F_damper : Outport  Port=2
  z_wheel : Outport  Port=3
  P_damper : Outport  Port=4
  wires:
  spring/2(z_wheel) -> z_wheel/1
  spring/1(Fz_spring) -> Bus Selector/1
  arb/1(F_arb) -> Bus Selector1/1
  Bus Selector/1 -> Add/1  "<Fz_spring_RF>"
  Bus Selector1/1 -> Add/2  "<Fz_arb_RF>"
  Bus Selector/2 -> Add1/1  "<Fz_spring_LF>"
  Bus Selector1/2 -> Add1/2  "<Fz_arb_LF>"
  Bus Selector/3 -> Add2/1  "<Fz_spring_RR>"
  Bus Selector1/3 -> Add2/2  "<Fz_arb_RR>"
  Bus Selector/4 -> Add3/1  "<Fz_spring_LR>"
  Bus Selector1/4 -> Add3/2  "<Fz_arb_LR>"
  Add/1 -> Bus Creator/1  "Fz_spring_RF"
  Add1/1 -> Bus Creator/2  "Fz_spring_LF"
  Add2/1 -> Bus Creator/3  "Fz_spring_RR"
  Add3/1 -> Bus Creator/4  "Fz_spring_LR"
  Bus Creator/1 -> F_spring/1
  z_wheel_vertical/1 -> spring/4(z_wheel_vert), damper/4(z_wheel_vert), arb/2(z_wheel_vert)
  z_body_vertical/1 -> damper/3(z_body_vert), spring/3(z_vert)
  z_body_pitch/1 -> damper/2(z_pitch), spring/2(z_pitch)
  z_body_roll/1 -> damper/1(z_roll), arb/1(z_roll), spring/1(z_roll)
  damper/1(F_damper) -> F_damper/1
  damper/2(P_damper) -> P_damper/1

== system body_chassis_vert/body_chassis_vert/transformation ==
  ax : Inport
  ay : Inport  Port=2
  vx : Inport  Port=3
  vy : Inport  Port=4
  az : Inport  Port=5
  vz : Inport  Port=6
  Bus Creator1 : BusCreator  Inputs=3
  Bus Creator2 : BusCreator  Inputs=3
  axyz : Outport
  vxyz : Outport  Port=2
  wires:
  vz/1 -> Bus Creator2/3  "vz"
  Bus Creator2/1 -> vxyz/1
  vy/1 -> Bus Creator2/2  "vy"
  vx/1 -> Bus Creator2/1  "vx"
  az/1 -> Bus Creator1/3  "az"
  Bus Creator1/1 -> axyz/1
  ay/1 -> Bus Creator1/2  "ay"
  ax/1 -> Bus Creator1/1  "ax"

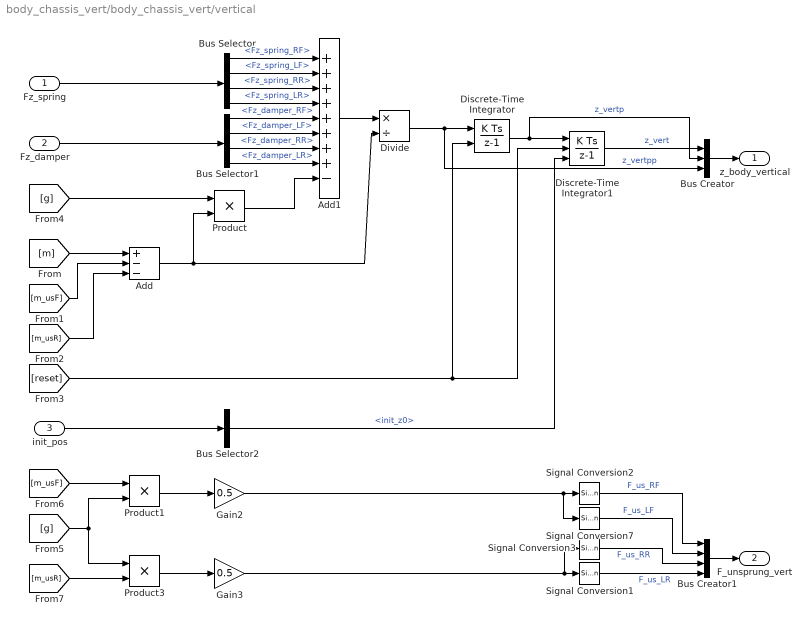
== system body_chassis_vert/body_chassis_vert/vertical ==
  Fz_spring : Inport
  Fz_damper : Inport  Port=2
  init_pos : Inport  Port=3
  Add : Sum  Inputs=+--
  Add1 : Sum  Inputs=++++++++-
  Bus Creator : BusCreator  Inputs=3
  Bus Creator1 : BusCreator  Inputs=4
  Bus Selector : BusSelector  OutputSignals=Fz_spring_RF,Fz_spring_LF,Fz_spring_RR,Fz_spring_LR
  Bus Selector1 : BusSelector  OutputSignals=Fz_damper_RF,Fz_damper_LF,Fz_damper_RR,Fz_damper_LR
  Bus Selector2 : BusSelector  OutputSignals=init_z0
  Discrete-Time Integrator : DiscreteIntegrator  ExternalReset=sampled level  SampleTime=-1  ICPrevOutput=DiscIntNeverNeededParam  ICPrevScaledInput=DiscIntNeverNeededParam
  Discrete-Time Integrator1 : DiscreteIntegrator  ExternalReset=sampled level  InitialConditionSource=external  SampleTime=-1  ICPrevOutput=DiscIntNeverNeededParam  ICPrevScaledInput=DiscIntNeverNeededParam
  Divide : Product  Inputs=*/
  Gain2 : Gain  Gain=0.5
  Gain3 : Gain  Gain=0.5
  Product : Product  RndMeth=Zero
  Product1 : Product  RndMeth=Zero
  Product3 : Product  RndMeth=Zero
  Signal Conversion{1..3,7} (4 alike) : SignalConversion  OverrideOpt=off
  z_body_vertical : Outport
  F_unsprung_vert : Outport  Port=2
  wires:
  [g] -> Product/1
  Add1/1 -> Divide/1
  Product/1 -> Add1/9
  init_pos/1 -> Bus Selector2/1
  Bus Selector2/1 -> Discrete-Time Integrator1/3  "<init_z0>"
  [reset] -> Discrete-Time Integrator1/2, Discrete-Time Integrator/2
  Bus Selector1/4 -> Add1/8  "<Fz_damper_LR>"
  Bus Selector1/3 -> Add1/7  "<Fz_damper_RR>"
  Bus Selector1/2 -> Add1/6  "<Fz_damper_LF>"
  Bus Selector1/1 -> Add1/5  "<Fz_damper_RF>"
  Bus Selector/4 -> Add1/4  "<Fz_spring_LR>"
  Bus Selector/3 -> Add1/3  "<Fz_spring_RR>"
  Bus Selector/2 -> Add1/2  "<Fz_spring_LF>"
  Bus Selector/1 -> Add1/1  "<Fz_spring_RF>"
  Fz_damper/1 -> Bus Selector1/1
  Fz_spring/1 -> Bus Selector/1
  Discrete-Time Integrator1/1 -> Bus Creator/1  "z_vert"
  Bus Creator/1 -> z_body_vertical/1
  Divide/1 -> Bus Creator/3, Discrete-Time Integrator/1  "z_vertpp"
  Discrete-Time Integrator/1 -> Bus Creator/2, Discrete-Time Integrator1/1  "z_vertp"
  Add/1 -> Divide/2, Product/2
  [m_usR] -> Add/3
  [m_usF] -> Add/2
  [m] -> Add/1
  [m_usF] -> Product1/1
  [g] -> Product3/1, Product1/2
  [m_usR] -> Product3/2
  Product1/1 -> Gain2/1
  Product3/1 -> Gain3/1
  Bus Creator1/1 -> F_unsprung_vert/1
  Signal Conversion7/1 -> Bus Creator1/2  "F_us_LF"
  Signal Conversion1/1 -> Bus Creator1/4  "F_us_LR"
  Gain2/1 -> Signal Conversion7/1, Signal Conversion2/1
  Signal Conversion2/1 -> Bus Creator1/1  "F_us_RF"
  Gain3/1 -> Signal Conversion3/1, Signal Conversion1/1
  Signal Conversion3/1 -> Bus Creator1/3  "F_us_RR"

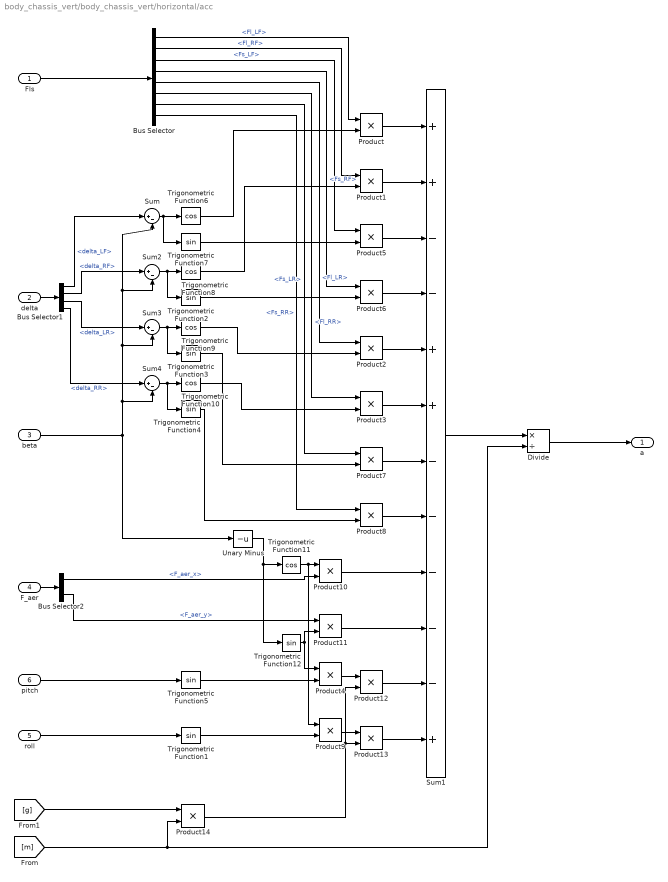
== system body_chassis_vert/body_chassis_vert/horizontal/acc ==
  Fls : Inport
  delta : Inport  Port=2
  beta : Inport  Port=3
  F_aer : Inport  Port=4
  roll : Inport  Port=5
  pitch : Inport  Port=6
  Bus Selector : BusSelector  OutputSignals=Fl.Fl_LF,Fl.Fl_RF,Fs.Fs_LF,Fs.Fs_RF,Fl.Fl_LR,Fl.Fl_RR,Fs.Fs_LR,Fs.Fs_RR
  Bus Selector1 : BusSelector  OutputSignals=delta_LF,delta_RF,delta_LR,delta_RR
  Bus Selector2 : BusSelector  OutputSignals=F_aer_x,F_aer_y
  Divide : Product  Inputs=*/
  Product{,1..14} (15 alike) : Product  RndMeth=Zero
  Sum{,2..4} (4 alike) : Sum  Inputs=|+-
  Sum1 : Sum  Inputs=++--++-----+
  Trigonometric Function{1..5,7,12} (7 alike) : Trigonometry
  Trigonometric Function{6,8..11} (5 alike) : Trigonometry  Operator=cos
  Unary Minus : UnaryMinus
  a : Outport
  wires:
  roll/1 -> Trigonometric Function1/1
  pitch/1 -> Trigonometric Function5/1
  [g] -> Product14/1
  Product9/1 -> Product13/1
  Trigonometric Function1/1 -> Product9/2
  Product14/1 -> Product12/2, Product13/2
  Product13/1 -> Sum1/12
  Product12/1 -> Sum1/11
  Product4/1 -> Product12/1
  Trigonometric Function5/1 -> Product4/2
  F_aer/1 -> Bus Selector2/1
  Unary Minus/1 -> Trigonometric Function11/1, Trigonometric Function12/1
  Trigonometric Function12/1 -> Product11/2, Product4/1
  Trigonometric Function11/1 -> Product10/1, Product9/1
  Bus Selector2/2 -> Product11/1  "<F_aer_y>"
  Bus Selector2/1 -> Product10/2  "<F_aer_x>"
  Product11/1 -> Sum1/10
  Trigonometric Function3/1 -> Product7/2
  Trigonometric Function10/1 -> Product3/2
  Sum4/1 -> Trigonometric Function4/1, Trigonometric Function10/1
  Sum3/1 -> Trigonometric Function3/1, Trigonometric Function9/1
  Sum2/1 -> Trigonometric Function2/1, Trigonometric Function8/1
  Sum1/1 -> Divide/1
  Product10/1 -> Sum1/9
  Product8/1 -> Sum1/8
  Product7/1 -> Sum1/7
  Product3/1 -> Sum1/6
  Trigonometric Function4/1 -> Product8/2
  Trigonometric Function9/1 -> Product2/2
  Product2/1 -> Sum1/5
  Product6/1 -> Sum1/4
  Product5/1 -> Sum1/3
  Product1/1 -> Sum1/2
  Product/1 -> Sum1/1
  Trigonometric Function2/1 -> Product6/2
  Trigonometric Function7/1 -> Product5/2
  Trigonometric Function8/1 -> Product1/2
  Trigonometric Function6/1 -> Product/2
  Sum/1 -> Trigonometric Function7/1, Trigonometric Function6/1
  beta/1 -> Unary Minus/1, Sum4/2, Sum3/2, Sum2/2, Sum/2
  delta/1 -> Bus Selector1/1
  Fls/1 -> Bus Selector/1
  Divide/1 -> a/1
  Bus Selector/1 -> Product/1  "<Fl_LF>"
  Bus Selector/2 -> Product1/1  "<Fl_RF>"
  Bus Selector/3 -> Product5/1  "<Fs_LF>"
  Bus Selector/4 -> Product6/1  "<Fs_RF>"
  Bus Selector/5 -> Product2/1  "<Fl_LR>"
  Bus Selector/6 -> Product3/1  "<Fl_RR>"
  Bus Selector/7 -> Product7/1  "<Fs_LR>"
  Bus Selector/8 -> Product8/1  "<Fs_RR>"
  Bus Selector1/2 -> Sum2/1  "<delta_RF>"
  Bus Selector1/1 -> Sum/1  "<delta_LF>"
  Bus Selector1/3 -> Sum3/1  "<delta_LR>"
  Bus Selector1/4 -> Sum4/1  "<delta_RR>"
  [m] -> Divide/2, Product14/2

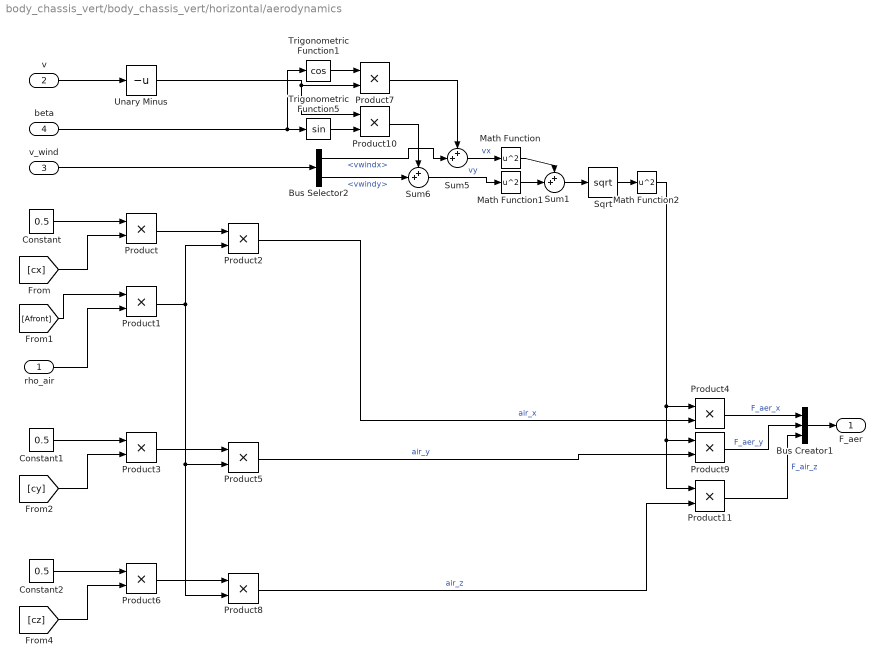
== system body_chassis_vert/body_chassis_vert/horizontal/aerodynamics ==
  rho_air : Inport
  v : Inport  Port=2
  v_wind : Inport  Port=3
  beta : Inport  Port=4
  Bus Creator1 : BusCreator  Inputs=3
  Bus Selector2 : BusSelector  OutputSignals=vwindx,vwindy
  Constant : Constant  Value=0.5
  Constant1 : Constant  Value=0.5
  Constant2 : Constant  Value=0.5
  Math Function : Math  Operator=square  SaturateOnIntegerOverflow=on
  Math Function1 : Math  Operator=square  SaturateOnIntegerOverflow=on
  Math Function2 : Math  Operator=square  SaturateOnIntegerOverflow=on
  Product{,1..11} (12 alike) : Product  RndMeth=Zero
  Sqrt : Sqrt  SaturateOnIntegerOverflow=on
  Sum1 : Sum  Inputs=++|
  Sum5 : Sum  Inputs=++|
  Sum6 : Sum  Inputs=++|
  Trigonometric Function1 : Trigonometry  Operator=cos
  Trigonometric Function5 : Trigonometry
  Unary Minus : UnaryMinus
  F_aer : Outport
  wires:
  Unary Minus/1 -> Product10/1, Product7/2
  Product11/1 -> Bus Creator1/3  "F_air_z"
  Math Function2/1 -> Product9/1, Product11/1, Product4/1
  Sqrt/1 -> Math Function2/1
  Sum1/1 -> Sqrt/1
  Math Function/1 -> Sum1/1
  Math Function1/1 -> Sum1/2
  Product7/1 -> Sum5/1
  Product10/1 -> Sum6/1
  v/1 -> Unary Minus/1
  Trigonometric Function1/1 -> Product7/1
  Trigonometric Function5/1 -> Product10/2
  Bus Creator1/1 -> F_aer/1
  Product9/1 -> Bus Creator1/2  "F_aer_y"
  Product4/1 -> Bus Creator1/1  "F_aer_x"
  Sum6/1 -> Math Function1/1  "vy"
  Sum5/1 -> Math Function/1  "vx"
  Bus Selector2/1 -> Sum5/2  "<vwindx>"
  Bus Selector2/2 -> Sum6/2  "<vwindy>"
  beta/1 -> Trigonometric Function1/1, Trigonometric Function5/1
  v_wind/1 -> Bus Selector2/1
  Product8/1 -> Product11/2  "air_z"
  Product6/1 -> Product8/1
  [cz] -> Product6/2
  Constant2/1 -> Product6/1
  Product5/1 -> Product9/2  "air_y"
  Product3/1 -> Product5/1
  [cy] -> Product3/2
  Constant1/1 -> Product3/1
  Product2/1 -> Product4/2  "air_x"
  Product1/1 -> Product8/2, Product5/2, Product2/2
  Product/1 -> Product2/1
  rho_air/1 -> Product1/2
  [Afront] -> Product1/1
  [cx] -> Product/2
  Constant/1 -> Product/1

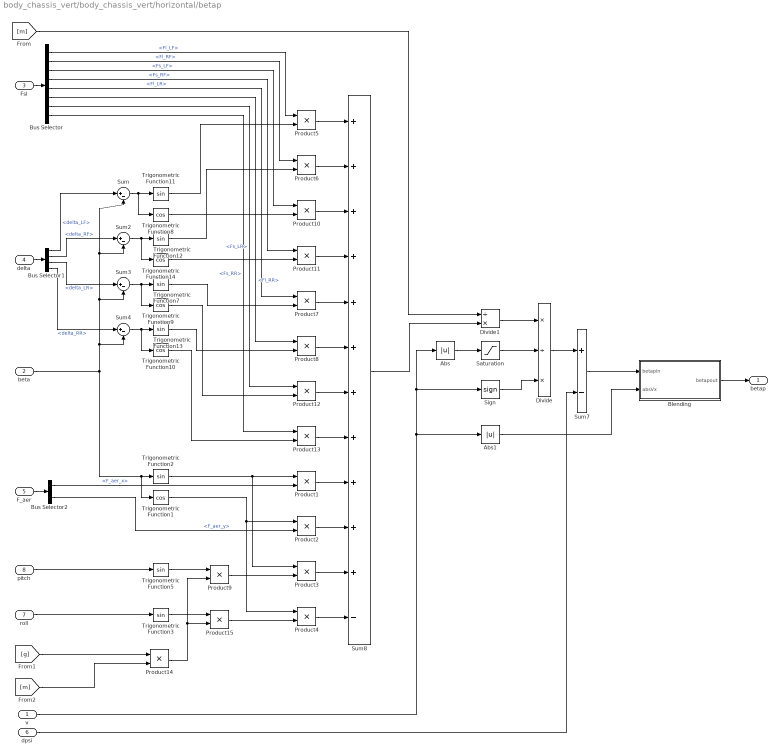
== system body_chassis_vert/body_chassis_vert/horizontal/betap ==
  v : Inport
  beta : Inport  Port=2
  Fsl : Inport  Port=3
  delta : Inport  Port=4
  F_aer : Inport  Port=5
  dpsi : Inport  Port=6
  roll : Inport  Port=7
  pitch : Inport  Port=8
  Abs : Abs
  Abs1 : Abs
  Blending : Subsystem
  Bus Selector : BusSelector  OutputSignals=Fl.Fl_LF,Fl.Fl_RF,Fs.Fs_LF,Fs.Fs_RF,Fl.Fl_LR,Fl.Fl_RR,Fs.Fs_LR,Fs.Fs_RR
  Bus Selector1 : BusSelector  OutputSignals=delta_LF,delta_RF,delta_LR,delta_RR
  Bus Selector2 : BusSelector  OutputSignals=F_aer_x,F_aer_y
  Divide : Product  Inputs=*/*
  Divide1 : Product  Inputs=/*
  Product{1..15} (15 alike) : Product  RndMeth=Zero
  Saturation : Saturate  UpperLimit=1e10  LowerLimit=0.5e-5
  Sign : Signum
  Sum{,2..4} (4 alike) : Sum  Inputs=|+-
  Sum7 : Sum  Inputs=+-
  Sum8 : Sum  Inputs=+++++++++++-
  Trigonometric Function{1,8..10,14} (5 alike) : Trigonometry  Operator=cos
  Trigonometric Function{2..3,5,7,11..13} (7 alike) : Trigonometry
  betap : Outport
  wires:
  roll/1 -> Trigonometric Function3/1
  pitch/1 -> Trigonometric Function5/1
  Product14/1 -> Product15/2, Product9/2
  Product15/1 -> Product4/2
  Product9/1 -> Product3/2
  Trigonometric Function3/1 -> Product15/1
  Trigonometric Function5/1 -> Product9/1
  [g] -> Product14/1
  [m] -> Product14/2
  Product4/1 -> Sum8/12
  Product3/1 -> Sum8/11
  Sign/1 -> Divide/3
  Sum7/1 -> Blending/1(betapin)
  Abs1/1 -> Blending/2(absVx)
  Abs/1 -> Saturation/1
  Trigonometric Function1/1 -> Product2/1, Product4/1
  Bus Selector2/2 -> Product2/2  "<F_aer_y>"
  Trigonometric Function2/1 -> Product1/1, Product3/1
  Bus Selector2/1 -> Product1/2  "<F_aer_x>"
  beta/1 -> Trigonometric Function1/1, Trigonometric Function2/1, Sum4/2, Sum3/2, Sum2/2, Sum/2
  Product2/1 -> Sum8/10
  F_aer/1 -> Bus Selector2/1
  Blending/1(betapout) -> betap/1
  v/1 -> Abs1/1, Sign/1, Abs/1
  Saturation/1 -> Divide/2
  Divide/1 -> Sum7/1
  dpsi/1 -> Sum7/2
  Trigonometric Function9/1 -> Product12/2
  Trigonometric Function13/1 -> Product8/2
  Sum4/1 -> Trigonometric Function13/1, Trigonometric Function10/1
  Sum3/1 -> Trigonometric Function7/1, Trigonometric Function9/1
  Sum2/1 -> Trigonometric Function14/1, Trigonometric Function12/1
  Sum8/1 -> Divide1/2
  Product1/1 -> Sum8/9
  Product13/1 -> Sum8/8
  Product12/1 -> Sum8/7
  Product8/1 -> Sum8/6
  Trigonometric Function10/1 -> Product13/2
  Trigonometric Function7/1 -> Product7/2
  Product7/1 -> Sum8/5
  Product11/1 -> Sum8/4
  Product10/1 -> Sum8/3
  Product6/1 -> Sum8/2
  Product5/1 -> Sum8/1
  Trigonometric Function14/1 -> Product11/2
  Trigonometric Function8/1 -> Product10/2
  Trigonometric Function12/1 -> Product6/2
  Trigonometric Function11/1 -> Product5/2
  Sum/1 -> Trigonometric Function11/1, Trigonometric Function8/1
  Divide1/1 -> Divide/1
  Bus Selector1/2 -> Sum2/1  "<delta_RF>"
  Bus Selector1/1 -> Sum/1  "<delta_LF>"
  Bus Selector1/3 -> Sum3/1  "<delta_LR>"
  Bus Selector1/4 -> Sum4/1  "<delta_RR>"
  delta/1 -> Bus Selector1/1
  Fsl/1 -> Bus Selector/1
  Bus Selector/1 -> Product5/1  "<Fl_LF>"
  Bus Selector/2 -> Product6/1  "<Fl_RF>"
  Bus Selector/3 -> Product10/1  "<Fs_LF>"
  Bus Selector/4 -> Product11/1  "<Fs_RF>"
  Bus Selector/5 -> Product7/1  "<Fl_LR>"
  Bus Selector/6 -> Product8/1  "<Fl_RR>"
  Bus Selector/7 -> Product12/1  "<Fs_LR>"
  Bus Selector/8 -> Product13/1  "<Fs_RR>"
  [m] -> Divide1/1

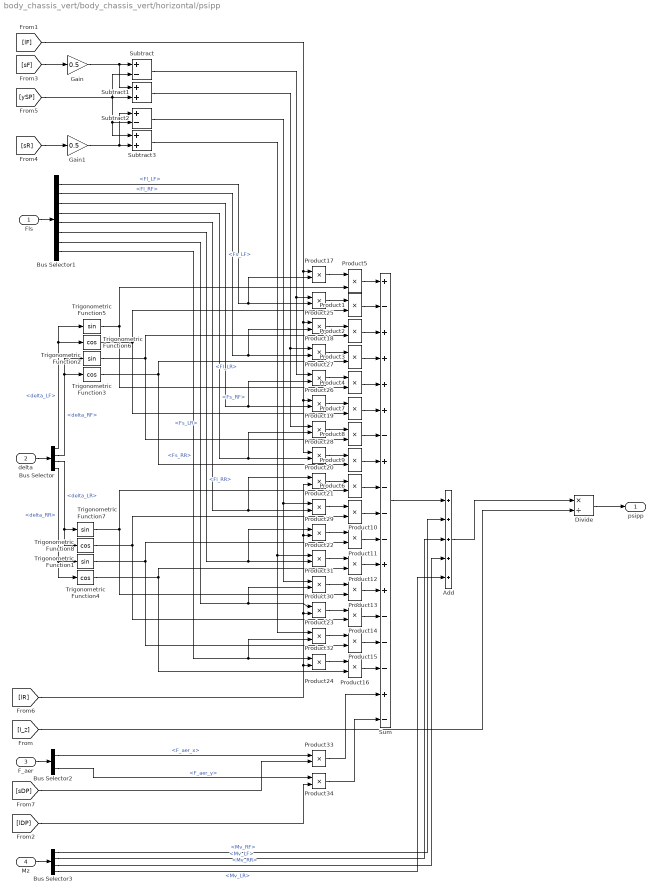
== system body_chassis_vert/body_chassis_vert/horizontal/psipp ==
  Fls : Inport
  delta : Inport  Port=2
  F_aer : Inport  Port=3
  Mz : Inport  Port=4
  Add : Sum  Inputs=5
  Bus Selector : BusSelector  OutputSignals=delta_LF,delta_RF,delta_LR,delta_RR
  Bus Selector1 : BusSelector  OutputSignals=Fl.Fl_LF,Fl.Fl_RF,Fs.Fs_LF,Fs.Fs_RF,Fl.Fl_LR,Fl.Fl_RR,Fs.Fs_LR,Fs.Fs_RR
  Bus Selector2 : BusSelector  OutputSignals=F_aer_x,F_aer_y
  Bus Selector3 : BusSelector  OutputSignals=Mv_RF,Mv_LF,Mv_RR,Mv_LR
  Divide : Product  Inputs=*/
  Gain : Gain  Gain=0.5
  Gain1 : Gain  Gain=0.5
  Product{1..34} (34 alike) : Product  RndMeth=Zero
  Subtract : Sum  Inputs=+-
  Subtract1 : Sum
  Subtract2 : Sum  Inputs=+-
  Subtract3 : Sum
  Sum : Sum  Inputs=+-++++-+---++---+-
  Trigonometric Function{1..2,5,7} (4 alike) : Trigonometry
  Trigonometric Function{3..4,6,8} (4 alike) : Trigonometry  Operator=cos
  psipp : Outport
  wires:
  Add/1 -> Divide/1
  Bus Selector3/1 -> Add/2  "<Mv_RF>"
  Bus Selector3/2 -> Add/3  "<Mv_LF>"
  Bus Selector3/3 -> Add/4  "<Mv_RR>"
  Bus Selector3/4 -> Add/5  "<Mv_LR>"
  Mz/1 -> Bus Selector3/1
  Sum/1 -> Add/1
  [lDP] -> Product34/2
  [sDP] -> Product33/2
  Product34/1 -> Sum/18
  Product33/1 -> Sum/17
  Bus Selector2/2 -> Product34/1  "<F_aer_y>"
  Bus Selector2/1 -> Product33/1  "<F_aer_x>"
  F_aer/1 -> Bus Selector2/1
  Bus Selector/2 -> Trigonometric Function2/1, Trigonometric Function3/1  "<delta_RF>"
  delta/1 -> Bus Selector/1
  Bus Selector/4 -> Trigonometric Function4/1, Trigonometric Function1/1  "<delta_RR>"
  Bus Selector/3 -> Trigonometric Function8/1, Trigonometric Function7/1  "<delta_LR>"
  Trigonometric Function4/1 -> Product16/2, Product12/2
  Trigonometric Function1/1 -> Product15/2, Product11/2
  Trigonometric Function8/1 -> Product14/2, Product10/2
  Trigonometric Function7/1 -> Product13/2, Product6/2
  Product24/1 -> Product16/1
  Product32/1 -> Product15/1
  Product23/1 -> Product14/1
  Product30/1 -> Product13/1
  Product16/1 -> Sum/16
  Product15/1 -> Sum/15
  Product14/1 -> Sum/14
  Product13/1 -> Sum/13
  Product12/1 -> Sum/12
  Product11/1 -> Sum/11
  Product10/1 -> Sum/10
  Product6/1 -> Sum/9
  Product31/1 -> Product12/1
  Product22/1 -> Product11/1
  Product29/1 -> Product10/1
  Product21/1 -> Product6/1
  Product20/1 -> Product9/1
  Product28/1 -> Product8/1
  Trigonometric Function3/1 -> Product9/2, Product3/2
  Product19/1 -> Product7/1
  Product26/1 -> Product4/1
  Product27/1 -> Product3/1
  Product18/1 -> Product2/1
  Trigonometric Function2/1 -> Product8/2, Product2/2
  Trigonometric Function6/1 -> Product7/2, Product1/2
  Trigonometric Function5/1 -> Product4/2, Product5/2
  Product9/1 -> Sum/8
  Product8/1 -> Sum/7
  Product7/1 -> Sum/6
  Product4/1 -> Sum/5
  Product3/1 -> Sum/4
  Product2/1 -> Sum/3
  Product25/1 -> Product1/1
  Product17/1 -> Product5/1
  Product1/1 -> Sum/2
  Product5/1 -> Sum/1
  Bus Selector1/8 -> Product24/1, Product32/2  "<Fs_RR>"
  Bus Selector1/6 -> Product22/1, Product31/2  "<Fl_RR>"
  Bus Selector1/5 -> Product21/1, Product29/2  "<Fl_LR>"
  Bus Selector/1 -> Trigonometric Function6/1, Trigonometric Function5/1  "<delta_LF>"
  Bus Selector1/4 -> Product20/2, Product28/2  "<Fs_RF>"
  Bus Selector1/3 -> Product19/2, Product26/2  "<Fs_LF>"
  Bus Selector1/1 -> Product17/2, Product25/2  "<Fl_LF>"
  Divide/1 -> psipp/1
  Bus Selector1/2 -> Product18/2, Product27/2  "<Fl_RF>"
  Bus Selector1/7 -> Product23/1, Product30/2  "<Fs_LR>"
  Fls/1 -> Bus Selector1/1
  [I_z] -> Divide/2
  [lF] -> Product20/1, Product19/1, Product18/1, Product17/1
  [lR] -> Product23/2, Product22/2, Product21/2, Product24/2
  [sF] -> Gain/1
  [ySP] -> Subtract1/2, Subtract/2, Subtract2/2, Subtract3/1
  Gain/1 -> Subtract/1, Subtract1/1
  [sR] -> Gain1/1
  Gain1/1 -> Subtract3/2, Subtract2/1
  Subtract/1 -> Product25/1, Product26/1
  Subtract1/1 -> Product27/1, Product28/1
  Subtract2/1 -> Product30/1, Product29/1
  Subtract3/1 -> Product32/1, Product31/1

== system body_chassis_vert/body_chassis_vert/horizontal/xy_kos ==
  dv : Inport
  v : Inport  Port=2
  beta : Inport  Port=3
  betap : Inport  Port=4
  psip : Inport  Port=5
  Product{,1..6} (7 alike) : Product  RndMeth=Zero
  Sum : Sum
  Sum1 : Sum  Inputs=-+
  Sum2 : Sum
  Trigonometric Function : Trigonometry  Operator=cos
  Trigonometric Function1 : Trigonometry
  ax : Outport
  ay : Outport  Port=2
  vx : Outport  Port=3
  vy : Outport  Port=4
  wires:
  Sum2/1 -> ay/1  "ay"
  Sum1/1 -> ax/1  "ax"
  Product/1 -> Sum2/1
  Product4/1 -> Sum2/2
  Product3/1 -> Sum1/1
  Product2/1 -> Sum1/2
  Product1/1 -> Product4/2, Product3/1
  Trigonometric Function1/1 -> Product3/2, Product/1, Product6/1
  Trigonometric Function/1 -> Product4/1, Product5/1, Product2/2
  dv/1 -> Product2/1, Product/2
  v/1 -> Product6/2, Product5/2, Product1/2
  Sum/1 -> Product1/1
  betap/1 -> Sum/1
  psip/1 -> Sum/2
  beta/1 -> Trigonometric Function1/1, Trigonometric Function/1
  Product6/1 -> vy/1  "vy"
  Product5/1 -> vx/1  "vx"
